simulink model "Two_compartment_linear"  (R2019b)
settings: Solver=VariableStepAuto  StartTime=0.0  StopTime=time  RelTol=1e-3
values from neighbouring files (symbols this model uses):
  breath = 60/f    (= 4)    [Model_simulation.m]
  E1 = 10    [Model_simulation.m]
  E2 = 10    [Model_simulation.m]
  E_th = 15    [Model_simulation.m]
  insptime = (ieratio(1)/(ieratio(1)+ieratio(2)))*100    [Model_simulation.m]
  Pcontrol = 5    [Model_simulation.m]
  PEEP = 5    [Model_simulation.m]
  R = 30    [Model_simulation.m]
  R1 = 5    [Model_simulation.m]
  R2 = 5    [Model_simulation.m]
  V0 = 2    [Model_simulation.m]
  V0_th = 4.6    [Model_simulation.m]
settings Model: Creator=Amne  LastModifiedBy=Amne
settings DataIOCC: ReturnWorkspaceOutputs=off
settings DebuggingCC: ArithmeticOperatorsInVariantConditions=warning
settings SFSimCC: SimUseLocalCustomCode=off  CustomCodeUndefinedFunction=UseInterfaceOnly
settings RTWCC: RTWUseLocalCustomCode=off

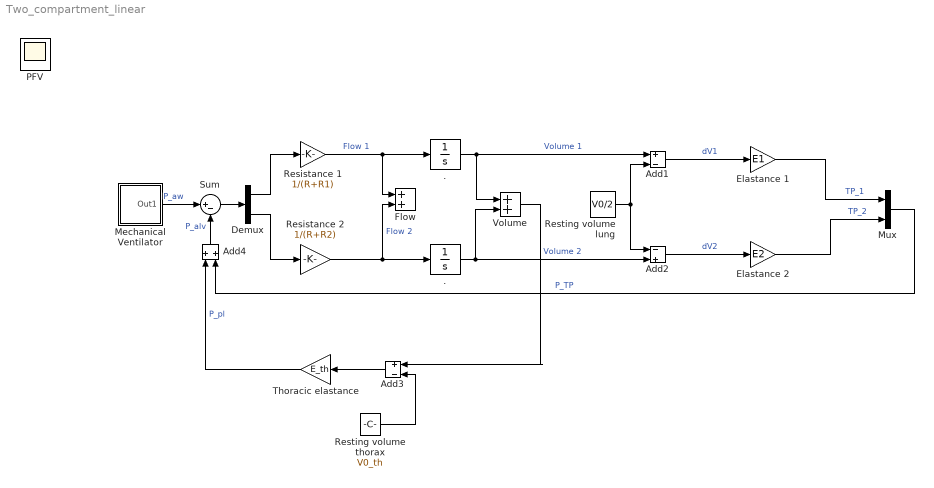
== system Two_compartment_linear ==
  " ." : Integrator  ZeroCross=off
  . : Integrator  ZeroCross=off
  Add1 : Sum  Inputs=+-
  Add2 : Sum  Inputs=-+
  Add3 : Sum  Inputs=+-
  Add4 : Sum
  Demux : Demux  Outputs=2
  Elastance 1 : Gain  Gain=E1
  Elastance 2 : Gain  Gain=E2
  "Flow " : Sum
  "Mechanical Ventilator " : Subsystem
  Mux : Mux  Inputs=2
  Resistance 1 : Gain  Gain=1/(R+R1)
  Resistance 2 : Gain  Gain=1/(R+R2)
  "Resting volume lung " : Constant  Value=V0/2
  Resting volume thorax : Constant  Value=V0_th
  Sum : Sum  Inputs=|+-
  Thoracic elastance : Gain  Gain=E_th
  "Volume " : Sum
  PFV : Scope
  wires:
  "Mechanical Ventilator "/1(Out1) -> Sum/1  "P_aw"
  Resistance 1/1 -> "Flow "/1, " ."/1  "Flow 1"
  " ."/1 -> "Volume "/1, Add1/1  "Volume 1"
  Resistance 2/1 -> "Flow "/2, ./1  "Flow 2"
  Sum/1 -> Demux/1
  Demux/1 -> Resistance 1/1
  Demux/2 -> Resistance 2/1
  Mux/1 -> Add4/2  "P_TP"
  ./1 -> "Volume "/2, Add2/2  "Volume 2"
  Resting volume thorax/1 -> Add3/2
  Add3/1 -> Thoracic elastance/1
  Thoracic elastance/1 -> Add4/1  "P_pl"
  Add4/1 -> Sum/2  "P_alv"
  "Resting volume lung "/1 -> Add1/2, Add2/1
  Add1/1 -> Elastance 1/1  "dV1"
  Add2/1 -> Elastance 2/1  "dV2"
  "Volume "/1 -> Add3/1
  Elastance 1/1 -> Mux/1  "TP_1"
  Elastance 2/1 -> Mux/2  "TP_2"

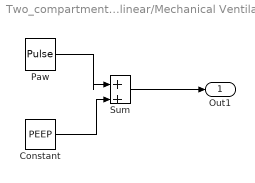
== system Two_compartment_linear/Mechanical Ventilator  ==
  Constant : Constant  Value=PEEP  SampleTime=0.1
  Paw : DiscretePulseGenerator  PulseType=Time based  Amplitude=Pcontrol  Period=breath  PulseWidth=insptime  PhaseDelay=2  SampleTime=0.1
  Sum : Sum  Inputs=|++
  Out1 : Outport  VectorParamsAs1DForOutWhenUnconnected=off
  wires:
  Paw/1 -> Sum/1
  Constant/1 -> Sum/2
  Sum/1 -> Out1/1
